simulink model "Drone_Formation"  (R2025a)
settings: Solver=FixedStepAuto  StartTime=0.0  StopTime=50  FixedStep=0.01  RelTol=1e-3
(part 2 of 2)

== matlab function Drone_Formation/Drone 3/Subsystem2/Uncontrolled_UAV1/Subsystem1/MATLAB Function ==
  data: tau input; phi_ddot output; phi_dot input; theta_dot input; psi_dot input; theta_ddot output; psi_ddot output; omega input
function [phi_ddot, theta_ddot, psi_ddot] = fcn(tau, phi_dot, theta_dot, psi_dot, omega)

    Ix = 4.8e-3; Iy = 4.8e-3; Iz = 9.8e-3;
    Jr = 1.287e-4;

    phi_ddot = (theta_dot*psi_dot*(Iy - Iz) - Jr*theta_dot*omega) + 1/Ix*tau(1);
    theta_ddot = (phi_dot*psi_dot*(Iz - Ix) + Jr*phi_dot*omega) + 1/Iy*tau(2);
    psi_ddot = (theta_dot*phi_dot*(Ix - Iy))/Iz + 1/Iz*tau(3);

end

== matlab function Drone_Formation/Drone 4/Subsystem2/MATLAB Function ==
  data: u input; force output; psi input; phi_r output; theta_r output
function [force, phi_r, theta_r] = fcn(u, psi)
    m = 1.5; g = 9.8;

    ux = u(1)*m;
    uy = u(2)*m;
    uz = (u(3)-g)*m;

    force = m*sqrt(ux^2 + uy^2 + (uz+g)^2);
    phi_r = asin(m*(ux*sin(psi) - uy*cos(psi))/force);
    theta_r = atan((ux*cos(psi) + uy*sin(psi))/(uz+g));
end

== matlab function Drone_Formation/Drone 1/Controller ==
  data: p_ref input; u output size=[3,1]; v_ref input; a_ref input; p input; v input; psi_r output
function [u, psi_r] = fcn(p_ref, v_ref, a_ref, p, v)

    kp = 4;
    kv = 3;

    A_adj = ones(5,5) - eye(5);
    a_ij = 0.5;

    L = zeros(5,5);
    for i = 1:5
        for j = 1:5
            if i ~= j && A_adj(i,j) == 1
                L(i,i) = L(i,i) + a_ij;
                L(i,j) = -a_ij;
            end
        end
    end

    psi_r = atan2(p_ref(2,1), p_ref(1,1));

    ep = p_ref(1:3,1) - p(1:3,1);
    ev = v_ref(1:3,1) - v(1:3,1);

    a = kron(L,ones(3))*((p_ref - p) + (v_ref - v));

    u = kp*ep + kv*ev + a_ref(1:3,1) + a(1:3,1);

end

== matlab function Drone_Formation/Drone 4/Subsystem2/MATLAB Function1 ==
  data: force input; w output; tau input; u output
function [w,u] = fcn(force, tau)

    l = 0.2; b = 2.92e-6; d = 1.12e-7;

    A = [b, b, b, b;
         0, -l*b, 0, l*b;
         -l*b, 0, l*b, 0;
         -d, d, -d, d];
    u = [force; tau(1); tau(2); tau(3)];
    w1 = A\u;
    w = sqrt(abs(w1));
    
end

== matlab function Drone_Formation/Drone 4/Subsystem2/MATLAB Function2 ==
  data: u input; y output
function y = fcn(u)
    
    y = u(1) + u(3) - u(2) - u(4);

end

== matlab function Drone_Formation/Drone 4/Subsystem2/Subsystem/Lower Control ==
  data: Q456 input size=3; tau_x output size=1; tau_y output size=1; tau_z output size=1; s456 input size=3
function [tau_x, tau_y, tau_z] = fcn(Q456, s456)

    Ix = 4.8e-3; Iy = 4.8e-3; Iz = 9.8e-3;
    a = 10;

    tau_x = Ix*(Q456(1) - 2*s456(1) - a*sign(s456(1)));
    tau_y = Iy*(Q456(2) - 2*s456(2) - a*sign(s456(2)));
    tau_z = Iz*(Q456(3) - 2*s456(3) - a*sign(s456(3)));

end

== matlab function Drone_Formation/Drone 4/Subsystem2/Subsystem/MATLAB Function ==
  data: angle_dot input; e_dot input size=3; e input size=3; Q456 output size=3; s456 output; omega input size=1; angle_r_ddot input size=3
function [Q456, s456] = fcn(angle_dot, e_dot, e, omega, angle_r_ddot)

    Ix = 4.8e-3; Iy = 4.8e-3; Iz = 9.8e-3;
    Jr = 1.287e-4;
    b = 10;

    Q456 = zeros(3,1);
    s456 = zeros(3,1);

    s456(1) = b*e(1) + e_dot(1);
    s456(2) = b*e(2) + e_dot(2);
    s456(3) = b*e(3) + e_dot(3);

    Q456(1) = -b*e_dot(1) + angle_r_ddot(1) - angle_dot(2)*angle_dot(3)*(Iy - Iz)/Ix - Jr*angle_dot(2)*omega/Ix;
    Q456(2) = -b*e_dot(2) + angle_r_ddot(2) - angle_dot(1)*angle_dot(3)*(Iz - Ix)/Iy + Jr*angle_dot(1)*omega/Iy;
    Q456(3) = -b*e_dot(3) + angle_r_ddot(3) - angle_dot(1)*angle_dot(2)*(Ix - Iy)/Iz;


end

== matlab function Drone_Formation/Drone 4/Subsystem2/Uncontrolled_UAV1/MATLAB Function1 ==
  data: force output; w1 input; w2 input; w3 input; w4 input; tau_x output; tau_y output; tau_z output; omega output
function [force, tau_x, tau_y, tau_z, omega] = fcn(w1, w2, w3, w4)

    l = 0.2; b = 2.92e-6; d = 1.12e-7;

    force = b*(w1^2 + w2^2 + w3^2 + w4^2);
    tau_x = l*b*(w4^2 - w2^2);
    tau_y = l*b*(w3^2 - w1^2);
    tau_z = d*(w2^2 + w4^2 - w1^2 - w3^2);
    omega = w1 + w3 - w2 - w4;

end

== matlab function Drone_Formation/Drone 4/Subsystem2/Uncontrolled_UAV1/Subsystem/MATLAB Function ==
  data: force input; x_ddot output; phi input; theta input; psi input; y_ddot output; z_ddot output
function [x_ddot, y_ddot, z_ddot] = fcn(force, phi, theta, psi)

    m = 1.5; g = 9.8;

    x_ddot = force*(cos(phi)*sin(theta)*cos(psi) + sin(phi)*sin(psi))/m;
    y_ddot = force*(cos(phi)*sin(theta)*sin(psi) - sin(phi)*cos(psi))/m;
    z_ddot = force*(cos(phi)*cos(theta))/m - g;

end

== matlab function Drone_Formation/Drone 4/Subsystem2/Uncontrolled_UAV1/Subsystem1/MATLAB Function ==
  data: tau input; phi_ddot output; phi_dot input; theta_dot input; psi_dot input; theta_ddot output; psi_ddot output; omega input
function [phi_ddot, theta_ddot, psi_ddot] = fcn(tau, phi_dot, theta_dot, psi_dot, omega)

    Ix = 4.8e-3; Iy = 4.8e-3; Iz = 9.8e-3;
    Jr = 1.287e-4;

    phi_ddot = (theta_dot*psi_dot*(Iy - Iz) - Jr*theta_dot*omega) + 1/Ix*tau(1);
    theta_ddot = (phi_dot*psi_dot*(Iz - Ix) + Jr*phi_dot*omega) + 1/Iy*tau(2);
    psi_ddot = (theta_dot*phi_dot*(Ix - Iy))/Iz + 1/Iz*tau(3);

end

== matlab function Drone_Formation/Drone 5/Subsystem2/MATLAB Function ==
  data: u input; force output; psi input; phi_r output; theta_r output
function [force, phi_r, theta_r] = fcn(u, psi)
    m = 1.5; g = 9.8;

    ux = u(1)*m;
    uy = u(2)*m;
    uz = (u(3)-g)*m;

    force = m*sqrt(ux^2 + uy^2 + (uz+g)^2);
    phi_r = asin(m*(ux*sin(psi) - uy*cos(psi))/force);
    theta_r = atan((ux*cos(psi) + uy*sin(psi))/(uz+g));
end

== matlab function Drone_Formation/Drone 5/Subsystem2/MATLAB Function1 ==
  data: force input; w output; tau input; u output
function [w,u] = fcn(force, tau)

    l = 0.2; b = 2.92e-6; d = 1.12e-7;

    A = [b, b, b, b;
         0, -l*b, 0, l*b;
         -l*b, 0, l*b, 0;
         -d, d, -d, d];
    u = [force; tau(1); tau(2); tau(3)];
    w1 = A\u;
    w = sqrt(abs(w1));
    
end

== matlab function Drone_Formation/Drone 5/Subsystem2/MATLAB Function2 ==
  data: u input; y output
function y = fcn(u)
    
    y = u(1) + u(3) - u(2) - u(4);

end

== matlab function Drone_Formation/Drone 5/Subsystem2/Subsystem/Lower Control ==
  data: Q456 input size=3; tau_x output size=1; tau_y output size=1; tau_z output size=1; s456 input size=3
function [tau_x, tau_y, tau_z] = fcn(Q456, s456)

    Ix = 4.8e-3; Iy = 4.8e-3; Iz = 9.8e-3;
    a = 10;

    tau_x = Ix*(Q456(1) - 2*s456(1) - a*sign(s456(1)));
    tau_y = Iy*(Q456(2) - 2*s456(2) - a*sign(s456(2)));
    tau_z = Iz*(Q456(3) - 2*s456(3) - a*sign(s456(3)));

end

== matlab function Drone_Formation/Drone 2/Subsystem/Kinematic ==
  data: p1_ddot output; u input
function p1_ddot = fcn(u)

    p1_ddot = u;

end

== matlab function Drone_Formation/Drone 5/Subsystem2/Subsystem/MATLAB Function ==
  data: angle_dot input; e_dot input size=3; e input size=3; Q456 output size=3; s456 output; omega input size=1; angle_r_ddot input size=3
function [Q456, s456] = fcn(angle_dot, e_dot, e, omega, angle_r_ddot)

    Ix = 4.8e-3; Iy = 4.8e-3; Iz = 9.8e-3;
    Jr = 1.287e-4;
    b = 10;

    Q456 = zeros(3,1);
    s456 = zeros(3,1);

    s456(1) = b*e(1) + e_dot(1);
    s456(2) = b*e(2) + e_dot(2);
    s456(3) = b*e(3) + e_dot(3);

    Q456(1) = -b*e_dot(1) + angle_r_ddot(1) - angle_dot(2)*angle_dot(3)*(Iy - Iz)/Ix - Jr*angle_dot(2)*omega/Ix;
    Q456(2) = -b*e_dot(2) + angle_r_ddot(2) - angle_dot(1)*angle_dot(3)*(Iz - Ix)/Iy + Jr*angle_dot(1)*omega/Iy;
    Q456(3) = -b*e_dot(3) + angle_r_ddot(3) - angle_dot(1)*angle_dot(2)*(Ix - Iy)/Iz;


end

== matlab function Drone_Formation/Drone 5/Subsystem2/Uncontrolled_UAV1/MATLAB Function1 ==
  data: force output; w1 input; w2 input; w3 input; w4 input; tau_x output; tau_y output; tau_z output; omega output
function [force, tau_x, tau_y, tau_z, omega] = fcn(w1, w2, w3, w4)

    l = 0.2; b = 2.92e-6; d = 1.12e-7;

    force = b*(w1^2 + w2^2 + w3^2 + w4^2);
    tau_x = l*b*(w4^2 - w2^2);
    tau_y = l*b*(w3^2 - w1^2);
    tau_z = d*(w2^2 + w4^2 - w1^2 - w3^2);
    omega = w1 + w3 - w2 - w4;

end

== matlab function Drone_Formation/Drone 5/Subsystem2/Uncontrolled_UAV1/Subsystem/MATLAB Function ==
  data: force input; x_ddot output; phi input; theta input; psi input; y_ddot output; z_ddot output
function [x_ddot, y_ddot, z_ddot] = fcn(force, phi, theta, psi)

    m = 1.5; g = 9.8;

    x_ddot = force*(cos(phi)*sin(theta)*cos(psi) + sin(phi)*sin(psi))/m;
    y_ddot = force*(cos(phi)*sin(theta)*sin(psi) - sin(phi)*cos(psi))/m;
    z_ddot = force*(cos(phi)*cos(theta))/m - g;

end

== matlab function Drone_Formation/Drone 5/Subsystem2/Uncontrolled_UAV1/Subsystem1/MATLAB Function ==
  data: tau input; phi_ddot output; phi_dot input; theta_dot input; psi_dot input; theta_ddot output; psi_ddot output; omega input
function [phi_ddot, theta_ddot, psi_ddot] = fcn(tau, phi_dot, theta_dot, psi_dot, omega)

    Ix = 4.8e-3; Iy = 4.8e-3; Iz = 9.8e-3;
    Jr = 1.287e-4;

    phi_ddot = (theta_dot*psi_dot*(Iy - Iz) - Jr*theta_dot*omega) + 1/Ix*tau(1);
    theta_ddot = (phi_dot*psi_dot*(Iz - Ix) + Jr*phi_dot*omega) + 1/Iy*tau(2);
    psi_ddot = (theta_dot*phi_dot*(Ix - Iy))/Iz + 1/Iz*tau(3);

end

== matlab function Drone_Formation/Drone 1/Controller based position ==
  data: p_ref input; u output size=[3,1]; v_ref input; a_ref input; p input; v input
function u = fcn(p_ref, v_ref, a_ref, p, v)

    kp = 4;
    kv = 3;

    A_adj = ones(5,5) - eye(5);
    a_ij = 0.5;

    L = zeros(5,5);
    for i = 1:5
        for j = 1:5
            if i ~= j && A_adj(i,j) == 1
                L(i,i) = L(i,i) + a_ij;
                L(i,j) = -a_ij;
            end
        end
    end

    ep = p_ref(1:3,1) - p(1:3,1);
    ev = v_ref(1:3,1) - v(1:3,1);

    a = kron(L,ones(3))*((p_ref - p) + (v_ref - v));

    u = kp*ep + kv*ev + a_ref(1:3,1) + a(1:3,1);

end

== matlab function Drone_Formation/Drone 2/MATLAB Function2 ==
  data: p_ref input; u output; v_ref input; a_ref input; p input; v input
function u = fcn(p_ref, v_ref, a_ref, p, v)

    kp = 4;
    kv = 3;

    A_adj = ones(5,5) - eye(5);
    a_ij = 0.5;

    L = zeros(5,5);
    for i = 1:5
        for j = 1:5
            if i ~= j && A_adj(i,j) == 1
                L(i,i) = L(i,i) + a_ij;
                L(i,j) = -a_ij;
            end
        end
    end

    ep = p_ref(4:6,1) - p(4:6,1);
    ev = v_ref(4:6,1) - v(4:6,1);

    a = kron(L,ones(3))*((p_ref - p) + (v_ref - v));

    u = kp*ep + kv*ev + a_ref(4:6,1) + a(4:6,1);

end

== matlab function Drone_Formation/Drone 2/MATLAB Function1 ==
  data: p_ref input; u output; v_ref input; a_ref input; p input; v input; psi_r output
function [u, psi_r] = fcn(p_ref, v_ref, a_ref, p, v)

    kp = 4;
    kv = 3;

    A_adj = ones(5,5) - eye(5);
    a_ij = 0.5;

    L = zeros(5,5);
    for i = 1:5
        for j = 1:5
            if i ~= j && A_adj(i,j) == 1
                L(i,i) = L(i,i) + a_ij;
                L(i,j) = -a_ij;
            end
        end
    end

    psi_r = atan2(p_ref(5,1), p_ref(4,1));

    ep = p_ref(4:6,1) - p(4:6,1);
    ev = v_ref(4:6,1) - v(4:6,1);

    a = kron(L,ones(3))*((p_ref - p) + (v_ref - v));

    u = kp*ep + kv*ev + a_ref(4:6,1) + a(4:6,1);

end

== matlab function Drone_Formation/Drone 3/MATLAB Function2 ==
  data: p_ref input; u output; v_ref input; a_ref input; p input; v input
function u = fcn(p_ref, v_ref, a_ref, p, v)

    kp = 4;
    kv = 3;

    A_adj = ones(5,5) - eye(5);
    a_ij = 0.5;

    L = zeros(5,5);
    for i = 1:5
        for j = 1:5
            if i ~= j && A_adj(i,j) == 1
                L(i,i) = L(i,i) + a_ij;
                L(i,j) = -a_ij;
            end
        end
    end


    ep = p_ref(7:9,1) - p(7:9,1);
    ev = v_ref(7:9,1) - v(7:9,1);

    a = kron(L,ones(3))*((p_ref - p) + (v_ref - v));

    u = kp*ep + kv*ev + a_ref(7:9,1) + a(7:9,1);

end

== matlab function Drone_Formation/Drone 4/MATLAB Function2 ==
  data: p_ref input; u output; v_ref input; a_ref input; p input; v input
function u = fcn(p_ref, v_ref, a_ref, p, v)

    kp = 4;
    kv = 3;

    A_adj = ones(5,5) - eye(5);
    a_ij = 0.5;

    L = zeros(5,5);
    for i = 1:5
        for j = 1:5
            if i ~= j && A_adj(i,j) == 1
                L(i,i) = L(i,i) + a_ij;
                L(i,j) = -a_ij;
            end
        end
    end


    ep = p_ref(10:12,1) - p(10:12,1);
    ev = v_ref(10:12,1) - v(10:12,1);

    a = kron(L,ones(3))*((p_ref - p) + (v_ref - v));

    u = kp*ep + kv*ev + a_ref(10:12,1) + a(10:12,1);

end

== matlab function Drone_Formation/Drone 5/MATLAB Function2 ==
  data: p_ref input; u output; v_ref input; a_ref input; p input; v input
function u = fcn(p_ref, v_ref, a_ref, p, v)

    kp = 4;
    kv = 3;

    A_adj = ones(5,5) - eye(5);
    a_ij = 0.5;

    L = zeros(5,5);
    for i = 1:5
        for j = 1:5
            if i ~= j && A_adj(i,j) == 1
                L(i,i) = L(i,i) + a_ij;
                L(i,j) = -a_ij;
            end
        end
    end

    ep = p_ref(13:15,1) - p(13:15,1);
    ev = v_ref(13:15,1) - v(13:15,1);

    a = kron(L,ones(3))*((p_ref - p) + (v_ref - v));

    u = kp*ep + kv*ev + a_ref(13:15,1) + a(13:15,1);

end

== matlab function Drone_Formation/Drone 3/Subsystem/Kinematic ==
  data: p1_ddot output; u input
function p1_ddot = fcn(u)

    p1_ddot = u;

end

== matlab function Drone_Formation/Drone 3/MATLAB Function1 ==
  data: p_ref input; u output; v_ref input; a_ref input; p input; v input; psi_r output
function [u, psi_r] = fcn(p_ref, v_ref, a_ref, p, v)

    kp = 4;
    kv = 3;

    A_adj = ones(5,5) - eye(5);
    a_ij = 0.5;

    L = zeros(5,5);
    for i = 1:5
        for j = 1:5
            if i ~= j && A_adj(i,j) == 1
                L(i,i) = L(i,i) + a_ij;
                L(i,j) = -a_ij;
            end
        end
    end

    psi_r = atan2(p_ref(8,1), p_ref(7,1));

    ep = p_ref(7:9,1) - p(7:9,1);
    ev = v_ref(7:9,1) - v(7:9,1);

    a = kron(L,ones(3))*((p_ref - p) + (v_ref - v));

    u = kp*ep + kv*ev + a_ref(7:9,1) + a(7:9,1);

end

== matlab function Drone_Formation/Drone 4/Subsystem/Kinematic ==
  data: p1_ddot output; u input
function p1_ddot = fcn(u)

    p1_ddot = u;

end

== matlab function Drone_Formation/Drone 4/MATLAB Function1 ==
  data: p_ref input; u output; v_ref input; a_ref input; p input; v input; psi_r output
function [u, psi_r] = fcn(p_ref, v_ref, a_ref, p, v)

    kp = 4;
    kv = 3;

    A_adj = ones(5,5) - eye(5);
    a_ij = 0.5;

    L = zeros(5,5);
    for i = 1:5
        for j = 1:5
            if i ~= j && A_adj(i,j) == 1
                L(i,i) = L(i,i) + a_ij;
                L(i,j) = -a_ij;
            end
        end
    end

    psi_r = atan2(p_ref(11,1), p_ref(10,1));

    ep = p_ref(10:12,1) - p(10:12,1);
    ev = v_ref(10:12,1) - v(10:12,1);

    a = kron(L,ones(3))*((p_ref - p) + (v_ref - v));

    u = kp*ep + kv*ev + a_ref(10:12,1) + a(10:12,1);

end
